simulink model "Drem_Grad"  (R2020a)
settings: Solver=VariableStepAuto  StartTime=0.0  StopTime=300  RelTol=1e-3
InitFcn:
  | Drem_Grad_varLoad
StopFcn:
  | traiettoria
values from neighbouring files (symbols this model uses):
  a = 2    [Drem_Grad_varLoad.m]
  b = 1    [Drem_Grad_varLoad.m]
  eMax = 0.1    [Drem_Grad_varLoad.m]
  eMean = 0.1    [Drem_Grad_varLoad.m]
  H = [h1;h2]    [Drem_Grad_varLoad.m]
  Lambda = tf([1 1],1)    [Drem_Grad_varLoad.m]
  s = tf('s')    [Drem_Grad_varLoad.m]
  thetaZero = [b0;a0]    [Drem_Grad_varLoad.m]
  W = minreal(alphas/Lambda)    [Drem_Grad_varLoad.m]
libraries: cstblocks x8, simulink x1
settings Model: Creator=alfystar  LastModifiedBy=gabriele

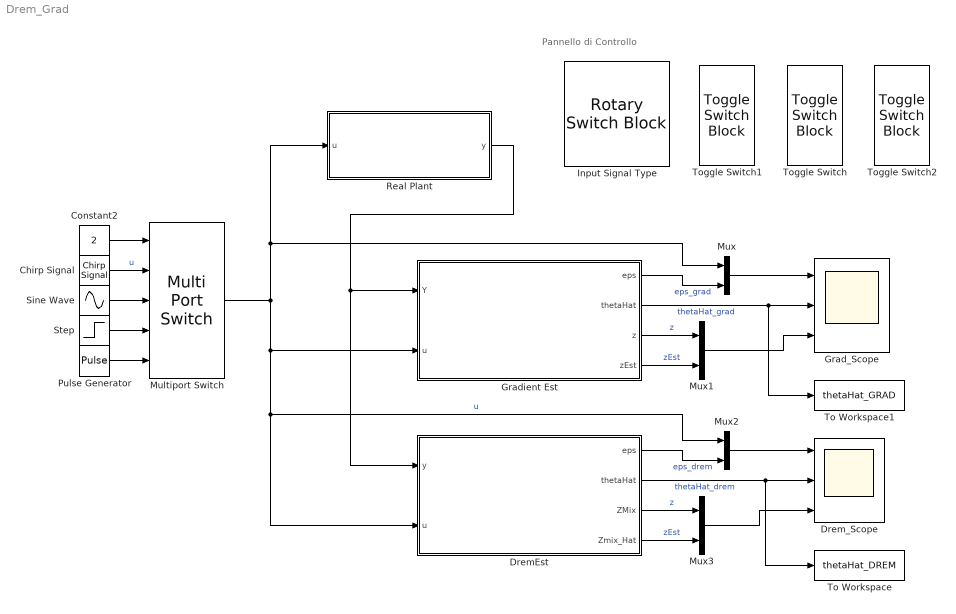
== system Drem_Grad ==
  note: Pannello di Controllo
  Chirp Signal : simulink/Sources/Chirp Signal  f1=0.1  T=100  f2=1
  Constant2 : Constant  Value=2
  DremEst : Subsystem
  Drem_Scope : Scope  NumInputPorts=3
  Grad_Scope : Scope  NumInputPorts=3
  Gradient Est : Subsystem
  Input Signal Type : RotarySwitchBlock  LabelPosition=Hide
      settings: Values={{'Chirp', 'Sine', 'Step', 'Impulse'}, [1 2 3 4]}
  Multiport Switch : MultiPortSwitch  DataPortOrder=Specify indices  DataPortIndices={1,2,3,4}
  Mux{,1..3} (4 alike) : Mux  Inputs=2
  Pulse Generator : DiscretePulseGenerator  PulseType=Time based  Amplitude=10  PulseWidth=5
  Real Plant : Subsystem
  Sine Wave : Sin  SampleTime=0
  Step : Step  SampleTime=0
  To Workspace : ToWorkspace  VariableName=thetaHat_DREM  SaveFormat=Timeseries  SampleTime=-1
  To Workspace1 : ToWorkspace  VariableName=thetaHat_GRAD  SaveFormat=Timeseries  SampleTime=-1
  Toggle Switch : ToggleSwitchBlock  LabelPosition=Hide
      settings: Values={{'Off_xNoise', 'On_xNoise'}, [0 1]}
  Toggle Switch1 : ToggleSwitchBlock  LabelPosition=Hide
      settings: Values={{'Off_uNoise', 'On_uNoise'}, [0 1]}
  Toggle Switch2 : ToggleSwitchBlock  LabelPosition=Hide
      settings: Values={{'Off_Prj', 'On_Prj'}, [1 2]}
  wires:
  Sine Wave/1 -> Multiport Switch/3
  Step/1 -> Multiport Switch/4
  Pulse Generator/1 -> Multiport Switch/5
  Chirp Signal/1 -> Multiport Switch/2  "u"
  Constant2/1 -> Multiport Switch/1
  Gradient Est/1(eps) -> Mux/2  "eps_grad"
  Gradient Est/2(thetaHat) -> To Workspace1/1, Grad_Scope/2  "thetaHat_grad"
  Mux/1 -> Grad_Scope/1
  Gradient Est/3(z) -> Mux1/1  "z"
  Gradient Est/4(zEst) -> Mux1/2  "zEst"
  Mux1/1 -> Grad_Scope/3
  Multiport Switch/1 -> Real Plant/1(u), Mux/1, Gradient Est/2(u), Mux2/1, DremEst/2(u)  "u"
  Mux3/1 -> Drem_Scope/3
  DremEst/3(ZMix) -> Mux3/1  "z"
  DremEst/1(eps) -> Mux2/2  "eps_drem"
  DremEst/2(thetaHat) -> To Workspace/1, Drem_Scope/2  "thetaHat_drem"
  Mux2/1 -> Drem_Scope/1
  DremEst/4(Zmix_Hat) -> Mux3/2  "zEst"
  Real Plant/1(y) -> Gradient Est/1(Y), DremEst/1(y)

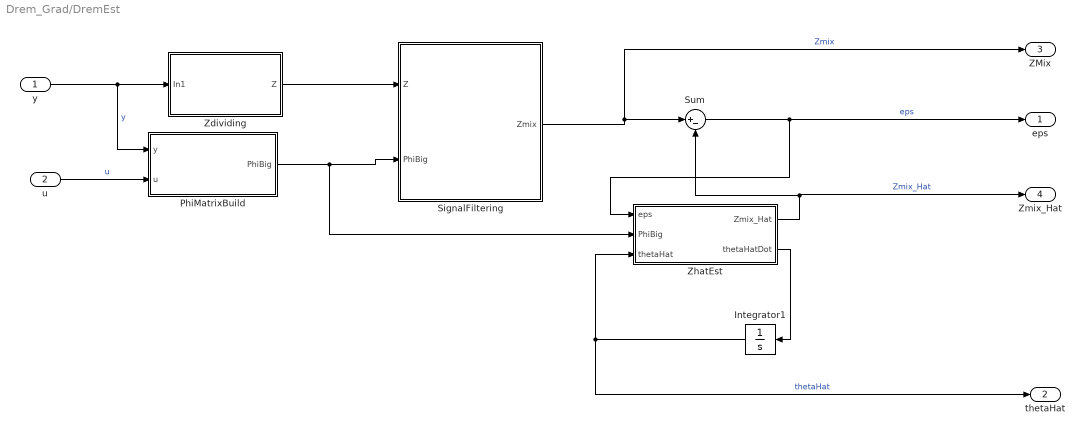
== system Drem_Grad/DremEst ==
  y : Inport
  u : Inport  Port=2
  Integrator1 : Integrator  InitialCondition=thetaZero
  PhiMatrixBuild : Subsystem
  SignalFiltering : MATLAB Function  TreatAsAtomicUnit=on
  Sum : Sum  Inputs=|+-
  Zdividing : Subsystem
  ZhatEst : MATLAB Function  TreatAsAtomicUnit=on
  eps : Outport
  thetaHat : Outport  Port=2
  ZMix : Outport  Port=3
  Zmix_Hat : Outport  Port=4
  wires:
  Sum/1 -> ZhatEst/1(eps), eps/1  "eps"
  Integrator1/1 -> thetaHat/1, ZhatEst/3(thetaHat)  "thetaHat"
  y/1 -> PhiMatrixBuild/1(y), Zdividing/1(In1)  "y"
  ZhatEst/1(Zmix_Hat) -> Zmix_Hat/1, Sum/2  "Zmix_Hat"
  SignalFiltering/1(Zmix) -> ZMix/1, Sum/1  "Zmix"
  Zdividing/1(Z) -> SignalFiltering/1(Z)
  PhiMatrixBuild/1(PhiBig) -> SignalFiltering/2(PhiBig), ZhatEst/2(PhiBig)
  u/1 -> PhiMatrixBuild/2(u)  "u"
  ZhatEst/2(thetaHatDot) -> Integrator1/1

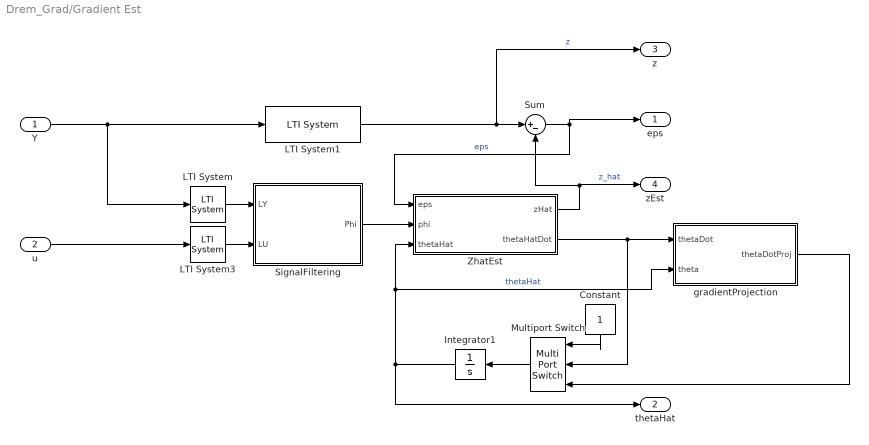
== system Drem_Grad/Gradient Est ==
  Y : Inport
  u : Inport  Port=2
  Constant : Constant
  Integrator1 : Integrator  InitialCondition=thetaZero
  LTI System : cstblocks/LTI System  sys=W  IC=[]
  LTI System1 : cstblocks/LTI System  sys=s/Lambda  IC=[]
  LTI System3 : cstblocks/LTI System  sys=W  IC=[]
  Multiport Switch : MultiPortSwitch  Inputs=2
  SignalFiltering : MATLAB Function  TreatAsAtomicUnit=on
  Sum : Sum  Inputs=|+-
  ZhatEst : MATLAB Function  TreatAsAtomicUnit=on
  gradientProjection : MATLAB Function  TreatAsAtomicUnit=on
  eps : Outport
  thetaHat : Outport  Port=2
  z : Outport  Port=3
  zEst : Outport  Port=4
  wires:
  SignalFiltering/1(Phi) -> ZhatEst/2(phi)
  Sum/1 -> ZhatEst/1(eps), eps/1  "eps"
  Integrator1/1 -> thetaHat/1, gradientProjection/2(theta), ZhatEst/3(thetaHat)  "thetaHat"
  LTI System1/1 -> z/1, Sum/1  "z"
  Y/1 -> LTI System1/1, LTI System/1
  u/1 -> LTI System3/1
  LTI System3/1 -> SignalFiltering/2(LU)
  LTI System/1 -> SignalFiltering/1(LY)
  ZhatEst/1(zHat) -> zEst/1, Sum/2  "z_hat"
  ZhatEst/2(thetaHatDot) -> Multiport Switch/2, gradientProjection/1(thetaDot)
  Multiport Switch/1 -> Integrator1/1
  Constant/1 -> Multiport Switch/1
  gradientProjection/1(thetaDotProj) -> Multiport Switch/3

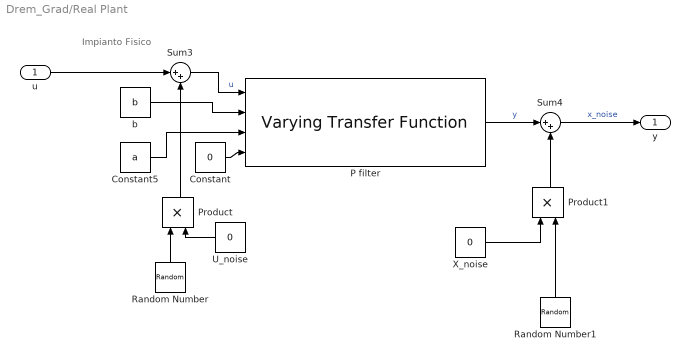
== system Drem_Grad/Real Plant ==
  note: Impianto Fisico
  u : Inport
  Constant : Constant  Value=0
  Constant5 : Constant  Value=a
  P filter : cstblocks/Linear Parameter Varying/Varying Transfer Function  N=1
  Product : Product
  Product1 : Product
  Random Number : RandomNumber  Mean=eMean  Variance=eMax  SampleTime=0.1
  Random Number1 : RandomNumber  Mean=eMean  Variance=eMax  SampleTime=0.1
  Sum3 : Sum  Inputs=|++
  Sum4 : Sum  Inputs=|++
  U_noise : Constant  Value=0
  X_noise : Constant  Value=0
  b : Constant  Value=b
  y : Outport
  wires:
  Random Number1/1 -> Product1/2
  P filter/1 -> Sum4/1  "y"
  Product/1 -> Sum3/2
  X_noise/1 -> Product1/1
  Sum4/1 -> y/1  "x_noise"
  Sum3/1 -> P filter/1  "u"
  Random Number/1 -> Product/1
  u/1 -> Sum3/1
  Product1/1 -> Sum4/2
  U_noise/1 -> Product/2
  Constant5/1 -> P filter/3
  Constant/1 -> P filter/4
  b/1 -> P filter/2

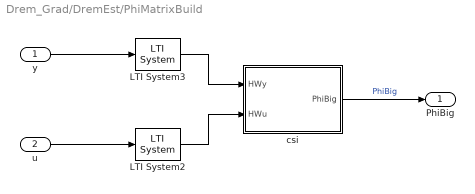
== system Drem_Grad/DremEst/PhiMatrixBuild ==
  y : Inport
  u : Inport  Port=2
  LTI System2 : cstblocks/LTI System  sys=H*W  IC=[]
  LTI System3 : cstblocks/LTI System  sys=H*W  IC=[]
  csi : MATLAB Function  TreatAsAtomicUnit=on
  PhiBig : Outport
  wires:
  csi/1(PhiBig) -> PhiBig/1  "PhiBig"
  y/1 -> LTI System3/1
  LTI System3/1 -> csi/1(HWy)
  LTI System2/1 -> csi/2(HWu)
  u/1 -> LTI System2/1

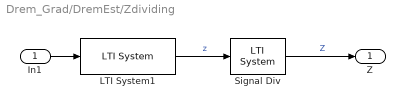
== system Drem_Grad/DremEst/Zdividing ==
  In1 : Inport
  LTI System1 : cstblocks/LTI System  sys=s/Lambda  IC=[]
  Signal Div : cstblocks/LTI System  sys=H  IC=[]
  Z : Outport
  wires:
  LTI System1/1 -> Signal Div/1  "z"
  Signal Div/1 -> Z/1  "Z"
  In1/1 -> LTI System1/1

== matlab function Drem_Grad/DremEst/SignalFiltering ==
  data: Z input; PhiBig input; Zmix output
function Zmix  = SignalMixing(Z,PhiBig)


Zmix = adjugate(PhiBig)*Z;

end

function B = adjugate(A)

% This finds the adjugate (adjoint) of square matrix A,
% and is valid even if A is singular or complex-valued.
% With u, s, and v obtained from [u,s,v] = svd(A), it
% makes use of the identity adj(A) = det(u*v')*v*adj(s)*u',
% which holds even if A and s are singular.  The expression,
% diag(prod(reshape(s0(ix),n-1,n),1)), accomplishes the
% evaluation of adj(s), each of whose diagonal elements
% is the product of all but one of the diagonal elements
% of s.  This requires that A be n x n where n >= 2.
% Roger Stafford - 10/18/06

[m,n] = size(A);
if (m ~= n) | (n < 2)
 error('Matrix A should be size n x n with n >= 2.')
end
[u,s,v] = svd(A);
s0 = diag(s);
ix = toeplitz(ones(n-1,1),[1 zeros(1,n-1)]) ...
     + repmat((1:n-1)',1,n);
B = det(u*v')*v*diag(prod(reshape(s0(ix),n-1,n),1))*u';

% ---
end

== matlab function Drem_Grad/DremEst/ZhatEst ==
  data: eps input; PhiBig input; thetaHat input; Zmix_Hat output; thetaHatDot output
function [Zmix_Hat, thetaHatDot] = Zhat(eps,PhiBig, thetaHat)

coder.extrinsic('evalin', 'assignin')
Gain = eye(2);                  % Needed in order to set variable class correctly
Gain = evalin('base','Gain'); % Read value from workspace

thetaHatDot = 10*Gain*det(PhiBig)*eps;
Zmix_Hat = thetaHat * det(PhiBig);
end

== matlab function Drem_Grad/Gradient Est/SignalFiltering ==
  data: LY input; LU input; Phi output
function Phi  = SignalFiltering(LY,LU)

Phi = [LU;
       -LY];

end

== matlab function Drem_Grad/Gradient Est/ZhatEst ==
  data: eps input; phi input; thetaHat input; zHat output; thetaHatDot output
function [zHat, thetaHatDot] = Zhat(eps,phi, thetaHat)

coder.extrinsic('evalin', 'assignin')
Gain = eye(2);                  % Needed in order to set variable class correctly
Gain = evalin('base','Gain'); % Read value from workspace

thetaHatDot = Gain*phi*eps;
zHat = thetaHat' * phi;
end

== matlab function Drem_Grad/DremEst/PhiMatrixBuild/csi ==
  data: HWy input; PhiBig output; HWu input
function PhiBig  = PhiMatrix(HWy,HWu)

PhiBig = [HWu -HWy];
end

== matlab function Drem_Grad/Gradient Est/gradientProjection ==
  data: thetaDot input; theta input; thetaDotProj output size=2
function thetaDotProj  = gradProject(thetaDot, theta)

coder.extrinsic('evalin', 'assignin')
Gain = eye(2);                  % Needed in order to set variable class correctly
Gain = evalin('base','Gain'); % Read value from workspace


% g(thetaHat) = [0; -theta2_hat] (= [0; -bHat])
%
% => Dg(thetaHat) = [0  0
%                    0 -1]

% thetaDotProj = thetaDot;
dg = [-2*theta(1) 0 ; 0 -1];

thetaDotProj = thetaDot;

g = gFunx(theta);
if ( all(g<0) || ( any(g==0) && all(all((thetaDot'*dg)<=0)) ) )
    return
end
fprintf("thetaDotProj perche fuori confine\n")
thetaDotProj = 1000*(thetaDot - Gain*dg*inv(dg'*Gain*dg)*dg'*Gain*thetaDot);


end

function v = gFunx(theta)
v = [-theta(1)^2;-theta(2)];
end
